simulink model "three_b_attitude_control_rotationMatrix"  (R2021a)
settings: Solver=ode23t  StartTime=0.0  StopTime=100  RelTol=1e-5
undefined symbols (not defined in the file): eul_init, g, I, km, kt, L, m, pm_0, sigbuilder_block, thrust_max, TQ_max_per_motor, Vb_init, Vm_0, wb_init, Xe_init, xme_0
libraries: simulink_extras x18, sharedtransform x3, simulink x1
(part 2 of 2)

== matlab function three_b_attitude_control_rotationMatrix/Control allocation and motor control/Ideal Actuators with allocation/Control allocation/FM_to_w2 ==
  data: L input; w2_cmd output; kt input; km input; Thrust input; M_x input; M_y input; M_z input
function w2_cmd = control_allocation(L, kt, km, Thrust, M_x, M_y, M_z)
%#codegen

    % construct the co-efficient matrix:
    %  F_and_M = C * w^2
    %
    % C = [
    %     kt  ,   kt   ,   kt  ,   kt  ;
    %     0   , -L*kt  ,   0   , L*kt  ;
    %    L*kt ,   0    , -L*kt ,   0   ;
    %     km ,   -km   ,  km  ,   -km  ;
    % ];

    % used Symbolic toolbox to compute inv(C)
%     C_inv = [
%                 1/(4*kt),          0 ,  1/(2*L*kt),  1/(4*km);
%                 1/(4*kt), -1/(2*L*kt),           0,  -1/(4*km); 
%                 1/(4*kt),          0 , -1/(2*L*kt),  1/(4*km);
%                 1/(4*kt), 1/(2*L*kt) ,          0 ,  -1/(4*km);
%              ];
         
    C_inv = [
             -1/(4*kt),            0,   1/(2*L*kt), -1/(4*km);
             -1/(4*kt),  -1/(2*L*kt),            0,  1/(4*km);
             -1/(4*kt),            0,  -1/(2*L*kt), -1/(4*km);
             -1/(4*kt),   1/(2*L*kt),            0,  1/(4*km);
            ];        
    % solve for the w^2 vec
    F_and_M_col = [Thrust, M_x, M_y, M_z].' ;

    w2_cmd = C_inv * F_and_M_col;
   
end

== matlab function three_b_attitude_control_rotationMatrix/Controllers/desired attitude ==
  data: phi_t input; bRg output; theta_t input; psi_t input
function bRg = calc_bRg(phi_t, theta_t,psi_t)
%#codegen

%    This function was generated by the Symbolic Math Toolbox version 8.7.
%    04-Nov-2022 08:55:57

bRg = reshape([cos(psi_t).*cos(theta_t),-cos(phi_t).*sin(psi_t)+cos(psi_t).*sin(phi_t).*sin(theta_t),sin(phi_t).*sin(psi_t)+cos(phi_t).*cos(psi_t).*sin(theta_t),cos(theta_t).*sin(psi_t),cos(phi_t).*cos(psi_t)+sin(phi_t).*sin(psi_t).*sin(theta_t),-cos(psi_t).*sin(phi_t)+cos(phi_t).*sin(psi_t).*sin(theta_t),-sin(theta_t),cos(theta_t).*sin(phi_t),cos(phi_t).*cos(theta_t)],[3,3]);

== matlab function three_b_attitude_control_rotationMatrix/Quad_EOM/Integrate_DCM/Calc Euler_rates/euler_rates ==
  data: phi_t input; euler_rates output; theta_t input; p input; q input; r input
function euler_rates = euler_rates(phi_t,theta_t,p,q,r)
%#codegen

%    This function was generated by the Symbolic Math Toolbox version 8.7.
%    04-Nov-2022 08:55:55

euler_rates = [(p.*cos(theta_t)+r.*cos(phi_t).*sin(theta_t)+q.*sin(phi_t).*sin(theta_t))./cos(theta_t);q.*cos(phi_t)-r.*sin(phi_t);(r.*cos(phi_t)+q.*sin(phi_t))./cos(theta_t)];

== matlab function three_b_attitude_control_rotationMatrix/Quad_EOM/Integrate_DCM/MATLAB Function ==
  data: w input; S output
function S = calc_S(w)
%#codegen

x = w(1);
y = w(2);
z = w(3);

S = [    0,  -z,   y;
         z,   0,  -x;
        -y,   x,   0;
    ];

== matlab function three_b_attitude_control_rotationMatrix/Quad_EOM/Integrate_DCM/MATLAB Function1 ==
  data: old_gRb input; new_gRb output
function new_gRb = correct_gRb(old_gRb)
%#codegen

% The correction technique implementde here is the one described by 
% William Premerlani and Paul Bizard:
%   see:  https://wiki.paparazziuav.org/w/images/e/e5/DCMDraft2.pdf

row_1   = old_gRb(1,:);
row_2   = old_gRb(2,:);

% look at the error associted with row_1 and row_2 they are supposed to be 
% orthogonal, ie: their DOT product should be ZERO
e       = sum( row_1 .* row_2);

% distrubute the error across X and Y
new_row_1 = row_1  - (e/2)*row_2;
new_row_2 = row_2  - (e/2)*row_1;

% compute Z
new_row_3 = cross( new_row_1, new_row_2 );

% normlaize all rows so that their MAG is UNITY
%:  NOTE:  norm([3 4]) is 5
new_row_1 = new_row_1 / norm(new_row_1);
new_row_2 = new_row_2 / norm(new_row_2);
new_row_3 = new_row_3 / norm(new_row_3);

% assemble the NEW gRb matrix
new_gRb = [new_row_1; new_row_2; new_row_3];

end

== matlab function three_b_attitude_control_rotationMatrix/Quad_EOM/Integrate_DCM/MATLAB Function2 ==
  data: R input; phi output; theta output; psi output
function [phi,theta,psi] = euler_from_rot(R)
% Get Euler angles from rotation matrix (wolrd to body rotation matrix)
%NOTE:  this is bRg ... and NOT gRb

phi   = atan2(R(2,3),R(3,3));
theta = -asin(R(1,3));
psi   = atan2(R(1,2), R(1,1));
end

== matlab function three_b_attitude_control_rotationMatrix/Controllers/MATLAB Function ==
  data: S input; omega output
function omega = S2vec(S)
% Skew symmetric matrix to vector

% S = [    0,  -z,   y;
%          z,   0,  -x;
%         -y,   x,   0;
%     ];

omega = [S(3,2); S(1,3); S(2,1)];

== matlab function three_b_attitude_control_rotationMatrix/Control allocation and motor control/Ideal Actuators with allocation/Perfect actuators/Allocation matrix (motor speed to twist) ==
  data: L input; Thrust output; kt input; km input; w2_col input; M_x output; M_y output; M_z output
function [Thrust, M_x, M_y, M_z] = mixer(L, kt, km, w2_col)
%#codegen



    % construct the co-efficient matrix:
    %  T = C * w^2
    
%     C = [
%         kt  ,   kt   ,   kt  ,   kt  ;
%         0   , -L*kt  ,   0   , L*kt  ;
%        L*kt ,   0    , -L*kt ,   0   ;
%         km ,   -km   ,  km  ,   -km  ;
%     ];

    C = [
        -kt  ,   -kt  ,   -kt ,   -kt  ;
        0    , -L*kt   ,   0   , L*kt  ;
       L*kt ,   0    , -L*kt  ,   0   ;
        -km  ,   km   ,  -km  ,   km  ;
    ];

    % solve for the FM_col
    %   FM_col = [Thrust, M_x, M_y, M_z].' ;
    
    FM_col  =  C * w2_col;
    
    Thrust  =  FM_col(1);
    M_x     =  FM_col(2);
    M_y     =  FM_col(3);
    M_z     =  FM_col(4);
    
end
